simulink model "control"  (R2023a)
settings: Solver=VariableStepAuto  StartTime=0.0  StopTime=10.0  RelTol=1e-3
undefined symbols (not defined in the file or in its folder): Levenberg, Marquardt
libraries: robotcorelib x2, robotmaniplib x1, simulink x1
settings Model: Creator=mkris  LastModifiedBy=mkris

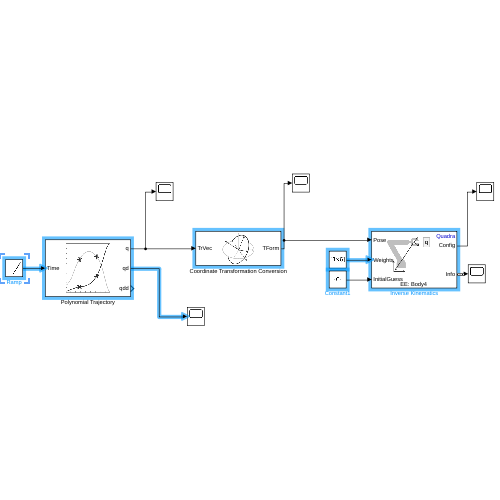
[thumbnail: Simulink's stored preview of the top-level diagram]
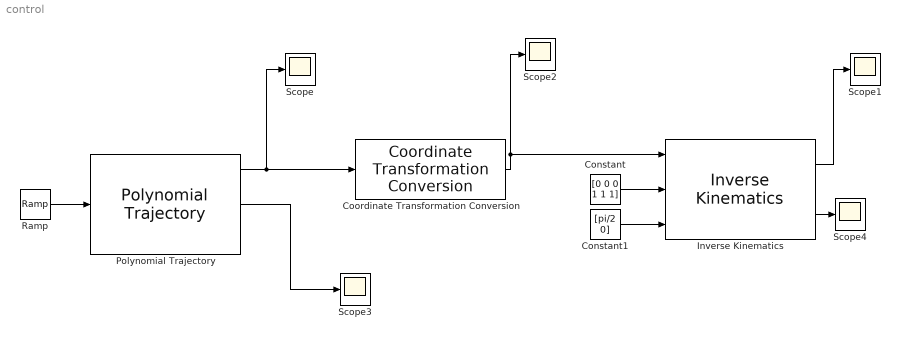
== system control ==
  Constant : Constant  Value=[0 0 0 1 1 1]  OutDataTypeStr=Inherit: Inherit via back propagation
  Constant1 : Constant  Value=[pi/2 0]  VectorParams1D=off
  Coordinate Transformation Conversion : robotcorelib/Coordinate Transformation Conversion  InputRepresentation=Translation Vector  InputEulerSequence=ZYX  ShowTrVecInputPort=on  OutputRepresentation=Homogeneous Transformation  OutputEulerSequence=ZYX  ShowTrVecOutputPort=on  SimulateUsing=Code generation
  Inverse Kinematics : robotmaniplib/Inverse Kinematics  RigidBodyTree=Quadra  EndEffector=Body4  ShowInfo=on  SolverName=Levenberg-Marquardt  EnforceJointLimits=off  MaxIterations=1500  MaxTime=10  GradientTolerance=1e-7  SolutionTolerance=1e-7  StepTolerance=1e-14  ErrorChangeTolerance=1e-12  UseErrorDamping=on  DampingBias=0.0025  SimulateUsing=Code generation
  Polynomial Trajectory : robotcorelib/Polynomial Trajectory  WaypointSource=Internal  Waypoints=[-1, 0, 1; -10.5, -9.5, -10.5; 5, 5, 5]  TimePoints=[ 0, 2.5, 5 ]  TimeInterval=[ 1, 4 ]  Method=Cubic Polynomial  ParameterSource=Internal  VelocityBoundaryCondition=zeros( 3, 3 )  AccelerationBoundaryCondition=zeros( 2, 5 )  SimulateUsing=Code generation
  Ramp : simulink/Sources/Ramp  slope=1  start=0  InitialOutput=0
  Scope{,1..4} (5 alike) : Scope
  wires:
  Coordinate Transformation Conversion/1 -> Inverse Kinematics/1, Scope2/1
  Ramp/1 -> Polynomial Trajectory/1
  Polynomial Trajectory/1 -> Scope/1, Coordinate Transformation Conversion/1
  Constant/1 -> Inverse Kinematics/2
  Constant1/1 -> Inverse Kinematics/3
  Inverse Kinematics/1 -> Scope1/1
  Polynomial Trajectory/2 -> Scope3/1
  Inverse Kinematics/2 -> Scope4/1
